simulink model "3-2"  (R2022b)
settings: Solver=VariableStepAuto  StartTime=0.0  StopTime=10.0  RelTol=1e-3
settings Model: Creator=Mavara-(Asus)  LastModifiedBy=Mavara-(Asus)

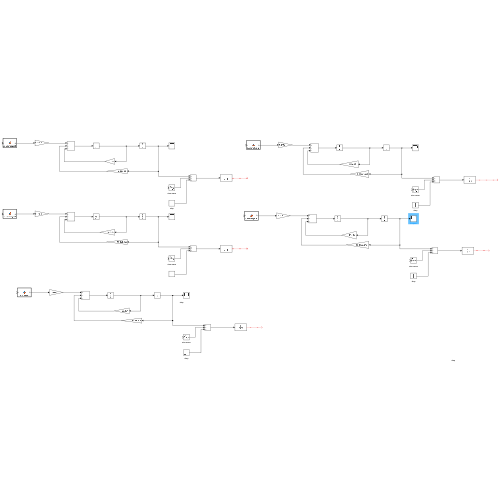
[thumbnail: Simulink's stored preview of the top-level diagram]
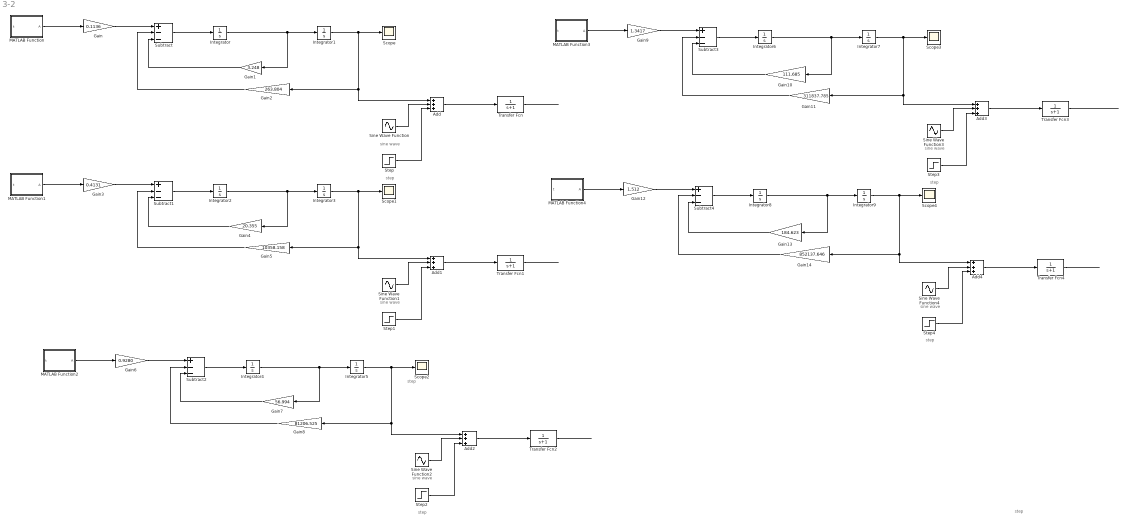
== system 3-2 ==
  note: step
  note: sine wave
  note: step
  note: sine wave
  note: step
  note: sine wave
  note: step
  note: sine wave
  note: step
  note: sine wave
  note: step
  Add{,1..4} (5 alike) : Sum  Inputs=+++
  Gain : Gain  Gain=0.1136
  Gain1 : Gain  Gain=3.248
  Gain10 : Gain  Gain=111.685
  Gain11 : Gain  Gain=311837.785
  Gain12 : Gain  Gain=1.512
  Gain13 : Gain  Gain=184.623
  Gain14 : Gain  Gain=852137.646
  Gain2 : Gain  Gain=263.804
  Gain3 : Gain  Gain=0.4131
  Gain4 : Gain  Gain=20.355
  Gain5 : Gain  Gain=10358.158
  Gain6 : Gain  Gain=0.9280
  Gain7 : Gain  Gain=56.994
  Gain8 : Gain  Gain=81206.525
  Gain9 : Gain  Gain=1.3417
  Integrator{,1..9} (10 alike) : Integrator
  MATLAB Function : MATLAB Function  TreatAsAtomicUnit=on
  MATLAB Function1 : MATLAB Function  TreatAsAtomicUnit=on
  MATLAB Function2 : MATLAB Function  TreatAsAtomicUnit=on
  MATLAB Function3 : MATLAB Function  TreatAsAtomicUnit=on
  MATLAB Function4 : MATLAB Function  TreatAsAtomicUnit=on
  Scope{,1..4} (5 alike) : Scope
  Sine Wave Function{,1..4} (5 alike) : Sin  TimeSource=Use external signal  SampleTime=0
  Step{,1..4} (5 alike) : Step  SampleTime=0
  Subtract{,1..4} (5 alike) : Sum  Inputs=+--
  Transfer Fcn{,1..4} (5 alike) : TransferFcn  Denominator=[1 1]
  wires:
  Gain10/1 -> Subtract3/3
  Step1/1 -> Add1/3
  Gain12/1 -> Subtract4/1
  Integrator7/1 -> Scope3/1, Add3/1, Gain11/1
  Step/1 -> Add/3
  Sine Wave Function4/1 -> Add4/2
  Integrator3/1 -> Scope1/1, Add1/1, Gain5/1
  Add4/1 -> Transfer Fcn4/1
  Add3/1 -> Transfer Fcn3/1
  Step4/1 -> Add4/3
  Subtract4/1 -> Integrator8/1
  Gain11/1 -> Subtract3/2
  Gain9/1 -> Subtract3/1
  Step3/1 -> Add3/3
  Gain7/1 -> Subtract2/3
  Integrator6/1 -> Gain10/1, Integrator7/1
  Gain14/1 -> Subtract4/2
  Gain1/1 -> Subtract/3
  Subtract2/1 -> Integrator4/1
  Sine Wave Function2/1 -> Add2/2
  Integrator4/1 -> Gain7/1, Integrator5/1
  Integrator5/1 -> Scope2/1, Add2/1, Gain8/1
  Gain2/1 -> Subtract/2
  Gain6/1 -> Subtract2/1
  Integrator9/1 -> Scope4/1, Add4/1, Gain14/1
  Gain5/1 -> Subtract1/2
  Integrator8/1 -> Gain13/1, Integrator9/1
  Sine Wave Function1/1 -> Add1/2
  Add1/1 -> Transfer Fcn1/1
  Gain3/1 -> Subtract1/1
  Integrator2/1 -> Gain4/1, Integrator3/1
  Add2/1 -> Transfer Fcn2/1
  Subtract3/1 -> Integrator6/1
  Step2/1 -> Add2/3
  Add/1 -> Transfer Fcn/1
  Integrator1/1 -> Scope/1, Add/1, Gain2/1
  Integrator/1 -> Gain1/1, Integrator1/1
  Sine Wave Function/1 -> Add/2
  Transfer Fcn4/1 -> ?
  Transfer Fcn3/1 -> ?
  Transfer Fcn/1 -> ?
  Subtract/1 -> Integrator/1
  Subtract1/1 -> Integrator2/1
  Transfer Fcn2/1 -> ?
  Gain4/1 -> Subtract1/3
  Gain8/1 -> Subtract2/2
  Transfer Fcn1/1 -> ?
  Gain13/1 -> Subtract4/3
  Sine Wave Function3/1 -> Add3/2
  Gain/1 -> Subtract/1
  MATLAB Function/1(A) -> Gain/1
  MATLAB Function1/1(A) -> Gain3/1
  MATLAB Function2/1(A) -> Gain6/1
  MATLAB Function3/1(A) -> Gain9/1
  MATLAB Function4/1(A) -> Gain12/1

== matlab function 3-2/MATLAB Function1 ==
  data: t input; A output
function A = customSignal(t)
    if t >= 0
        A = exp(3*t); % Since u(t) = 1 for t >= 0
    else
        A = 0; % Since u(t) = 0 for t < 0
    end
end

== matlab function 3-2/MATLAB Function2 ==
  data: t input; A output
function A = customSignal(t)
    if t >= 0
        A = exp(3*t); % Since u(t) = 1 for t >= 0
    else
        A = 0; % Since u(t) = 0 for t < 0
    end
end

== matlab function 3-2/MATLAB Function3 ==
  data: t input; A output
function A = customSignal(t)
    if t >= 0
        A = exp(3*t); % Since u(t) = 1 for t >= 0
    else
        A = 0; % Since u(t) = 0 for t < 0
    end
end

== matlab function 3-2/MATLAB Function4 ==
  data: t input; A output
function A = customSignal(t)
    if t >= 0
        A = exp(3*t); % Since u(t) = 1 for t >= 0
    else
        A = 0; % Since u(t) = 0 for t < 0
    end
end

== matlab function 3-2/MATLAB Function ==
  data: t input; A output
function A = customSignal(t)
    if t >= 0
        A = exp(3*t); % Since u(t) = 1 for t >= 0
    else
        A = 0; % Since u(t) = 0 for t < 0
    end
end
